simulink model "B737_PAH"  (R2018a)
settings: Solver=VariableStepAuto  StartTime=0.0  StopTime=S.simtime  RelTol=1e-3
undefined symbols (not defined in the file): S, sigbuilder_block
settings Model: Creator=Can Bekar  LastModifiedBy=Can Bekar
settings DataIOCC: ExternalInput=S.usignal  LoadExternalInput=on  SignalLogging=off  DSMLogging=off

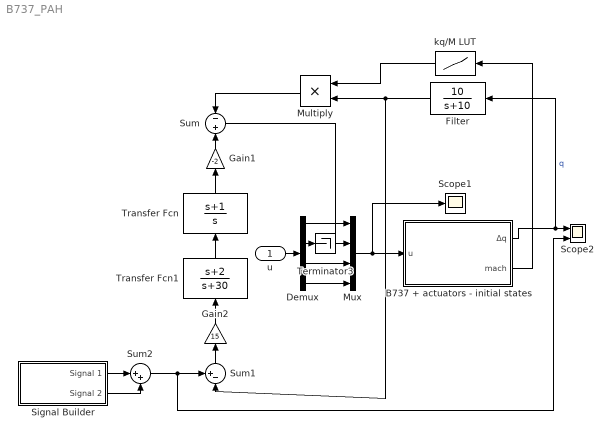
== system B737_PAH ==
  u : Inport
  B737 + actuators - initial states : Subsystem
  Demux : Demux
  Filter : TransferFcn  Numerator=[10]  Denominator=[1 10]
  Gain1 : Gain  Gain=-2
  Gain2 : Gain  Gain=15
  Multiply : Product
  Mux : Mux
  Scope1 : Scope
  Scope2 : Scope  NumInputPorts=2
  Signal Builder : Subsystem  Tag=STV Subsys  LoadFcn=sigbuilder_block('load');  StartFcn=sigbuilder_block('start');  StopFcn=sigbuilder_block('stop');  ClipboardFcn=sigbuilder_block('clipboard');  mask(Sigbuilder block){tuvar=[0:10]}
      mask help: Simulink:masks:SigbuilderBlock_MD
      mask init:
      | if ~strcmp(get_param(bdroot(gcbh),'SimulationStatus'),'stopped') tuvar = sigbuilder_block('maskInit'); end
      settings: CopyFcn=sigbuilder_block('copy');  DeleteFcn=sigbuilder_block('delete');  ModelCloseFcn=sigbuilder_block('modelClose');  PreSaveFcn=sigbuilder_block('preSave');  PauseFcn=sigbuilder_block('pause');  ContinueFcn=sigbuilder_block('continue');  NameChangeFcn=sigbuilder_block('namechange');  OpenFcn=sigbuilder_block('open',[233.25 91.5 964.5 399.75 ]);  CloseFcn=sigbuilder_block('close');
      mask Display: plot(0, 0, 100, 100,[2, 2, 32, 32, 2], [68, 8, 8, 68, 68],[32, 2], [38, 38], [32, 19, 2],[53, 60, 44], [32, 17, 17, 2],[16, 16, 31, 31]);txt = getActiveGroup(gcbh);text(2, 100, txt,'verticalAlignment', 'top');
  Sum : Sum  Inputs=-|+
  Sum1 : Sum  Inputs=+-|
  Sum2 : Sum  Inputs=|++
  Terminator3 : Terminator
  Transfer Fcn : TransferFcn  Numerator=[1 1]  Denominator=[1 0]
  Transfer Fcn1 : TransferFcn  Numerator=[1 2]  Denominator=[1 30]
  kq/M LUT : Lookup_n-D  NumberOfTableDimensions=1  BreakpointsForDimension1=S.M'  Table=S.kqLUT  InternalRulePriority=Speed  RndMeth=Simplest  InputSameDT=on
  wires:
  u/1 -> Demux/1
  Mux/1 -> Scope1/1, B737 + actuators - initial states/1(u)
  Demux/1 -> Mux/1
  Demux/3 -> Mux/3
  Demux/4 -> Mux/4
  B737 + actuators - initial states/1(Δq) -> Filter/1, Scope2/1  "q"
  Filter/1 -> Multiply/2, Sum1/2
  Multiply/1 -> Sum/1
  Transfer Fcn/1 -> Gain1/1
  Gain1/1 -> Sum/2
  Sum/1 -> Mux/2
  Signal Builder/2(Signal 2) -> Sum2/2
  Sum2/1 -> Scope2/2, Sum1/1
  Transfer Fcn1/1 -> Transfer Fcn/1
  Gain2/1 -> Transfer Fcn1/1
  Sum1/1 -> Gain2/1
  Signal Builder/1(Signal 1) -> Sum2/1
  Demux/2 -> Terminator3/1
  kq/M LUT/1 -> Multiply/1
  B737 + actuators - initial states/2(mach) -> kq/M LUT/1

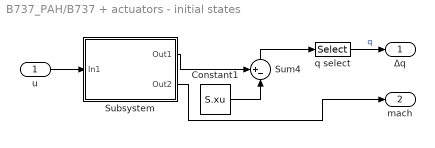
== system B737_PAH/B737 + actuators - initial states ==
  u : Inport
  Constant1 : Constant  Value=S.xu
  Subsystem : Subsystem
  Sum4 : Sum  Inputs=+-|
  q select : Selector  InputPortWidth=12  IndexOptions=Index vector (dialog)  Indices=[8]  OutputSizes=1
  Δq : Outport
  mach : Outport  Port=2
  wires:
  q select/1 -> Δq/1  "q"
  Sum4/1 -> q select/1
  Subsystem/1(Out1) -> Sum4/1
  u/1 -> Subsystem/1(In1)
  Constant1/1 -> Sum4/2
  Subsystem/2(Out2) -> mach/1

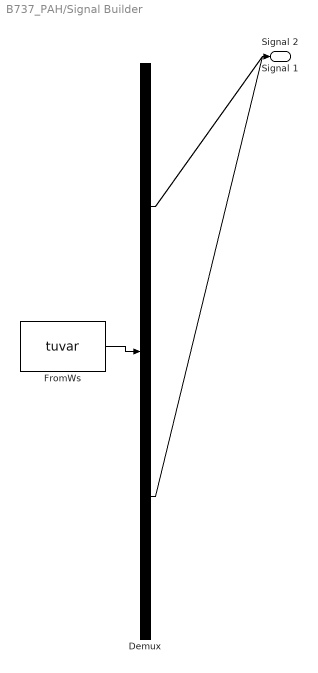
== system B737_PAH/Signal Builder ==
  Demux : Demux  Tag=STV Demux  Outputs=2
  FromWs : FromWorkspace  Tag=STV FromWs  VariableName=tuvar  SampleTime=0
      SigBuilderData=|
      | common.afterFinalStr = 'Extrapolate'
      | common.sampleTime = 0
      | dataSet.timeRange = [0 300]
      | dataSet.name = 'Group 1'
      | sbobj.Groups.Name = 'Group 1'
      | sbobj.Groups.Signals(1).Name = 'Signal 1'
      | sbobj.Groups.Signals(1).XData = [0 50 50 59.5 59.5 69 69 89 134.5 200 300]
      | sbobj.Groups.Signals(1).YData = [0 0 0.0041 0.0041 -0.0002 -0.0001 0.00165 0.00155 0.00155 -0.0001 0]
      | sbobj.Groups.Signals(2).Name = 'Signal 2'
      | sbobj.Groups.Signals(2).XData = [0 200 200 250.5 250.5 300]
      | sbobj.Groups.Signals(2).YData = [0 0 -0.0102 -0.0102 0 0]
      | sbobj.Groups.TimeRange = [0 300]
  Signal 1 : Outport  Tag=STV Outport
  Signal 2 : Outport  Tag=STV Outport  Port=2
  wires:
  FromWs/1 -> Demux/1
  Demux/1 -> Signal 1/1
  Demux/2 -> Signal 2/1

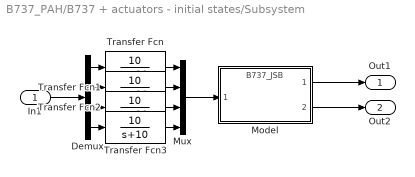
== system B737_PAH/B737 + actuators - initial states/Subsystem ==
  In1 : Inport
  Demux : Demux
  Model : ModelReference  ModelNameDialog=B737_JSB  SimulationMode=Normal  ModelReferenceVersion=1.187
  Mux : Mux
  Transfer Fcn{,1..3} (4 alike) : TransferFcn  Numerator=[10]  Denominator=[1 10]
  Out1 : Outport
  Out2 : Outport  Port=2
  wires:
  In1/1 -> Demux/1
  Model/1 -> Out1/1
  Mux/1 -> Model/1
  Transfer Fcn/1 -> Mux/1
  Demux/1 -> Transfer Fcn/1
  Demux/2 -> Transfer Fcn1/1
  Transfer Fcn1/1 -> Mux/2
  Demux/3 -> Transfer Fcn2/1
  Transfer Fcn2/1 -> Mux/3
  Demux/4 -> Transfer Fcn3/1
  Transfer Fcn3/1 -> Mux/4
  Model/2 -> Out2/1
